simulink model "s2"  (Simulink 2.00)
settings: Solver=ode5  StartTime=0.0  StopTime=tstop  FixedStep=0.005  MaxStep=0.005  RelTol=1e-6  AbsTol=1e-6
values from neighbouring files (symbols this model uses):
  alpha = input('Enter attenuation factor, alpha > ')    [M2.M]    (also in M3.M = input('Enter attenuation factor alpha, try 1,  > '))
  m = input('Enter value of m  > ')    [M2.M]    (also in M3.M = input('Enter the value of m for abc currents  > '))
  n = input('Enter value of harmonic order n  > ')    [M2.M]
undefined symbols (not defined in the file or in its folder): sfunxy
settings Model: SaveTime=off  SaveOutput=off  ConsistencyChecking=off

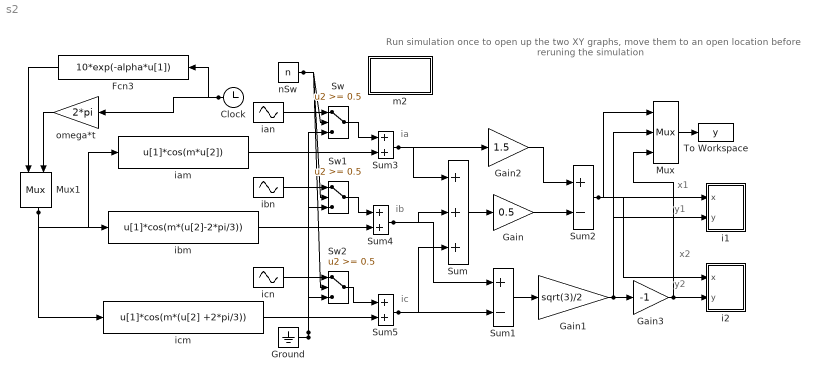
== system s2 ==
  note: ib
  note: ic
  note: x1
  note: x2
  note: y1
  note: y2
  note: ia
  note: Run simulation once to open up the two XY graphs, move
      | them to an open location before reruning  the simulation
  Clock : Clock
      settings: DeleteFcn=simclock BlockIsBeingDestroyed  PostSaveFcn=simclock Save
  Fcn3 : Fcn  Orientation=left  Expr=10*exp(-alpha*u[1])
  Gain : Gain  Gain=0.5
  Gain1 : Gain  Gain=sqrt(3)/2
  Gain2 : Gain  Gain=1.5
  Gain3 : Gain  Gain=-1
  Ground : Ground
  m2 : Subsystem
      settings: OpenFcn=m2
      mask Type: Masked block of m2.m
      mask Help: Uses m2.m to initialize and plot results
      mask Display: disp('Initialize\nand plot')
  Mux : Mux  Inputs=3
  Mux1 : Mux  Orientation=down  Inputs=2
  Sum : Sum  Inputs=+++
  Sum1 : Sum  Inputs=+-
  Sum2 : Sum  Inputs=+-
  Sum3 : Sum  Inputs=++
  Sum4 : Sum  Inputs=++
  Sum5 : Sum  Inputs=++
  Sw : Switch  Threshold=0.5
  Sw1 : Switch  Threshold=0.5
  Sw2 : Switch  Threshold=0.5
  To Workspace : ToWorkspace  VariableName=y  SampleTime=0
      settings: Buffer=1000
  i1 : Subsystem  mask(XY scope.){ax(1)=-20, ax(2)=20, ax(3)=-20, ax(4)=20, st=-1}
      mask prompts: ax(1) "x-min"; ax(2) "x-max"; ax(3) "y-min"; ax(4) "y-max"; st "Sample Time"
      mask help: XY scope using MATLAB graph window. First input is used as time base. Enter plotting ranges.
      mask Help: This block can be used to explore limit cycles. Look at the m-file sfunxy.m to see how it works.
      mask Display: plot([.05 .95 .95 .05 .05],[.45 .45 .95 .95 .45], 0.5+cos(0:0.1:2*pi)*0.3,0.7+sin(0:0.1:2*pi)*0.2)
  i2 : Subsystem  mask(XY scope.){ax(1)=-20, ax(2)=20, ax(3)=-20, ax(4)=20, st=-1}
      mask prompts: ax(1) "x-min"; ax(2) "x-max"; ax(3) "y-min"; ax(4) "y-max"; st "Sample Time"
      mask help: XY scope using MATLAB graph window. First input is used as time base. Enter plotting ranges.
      mask Help: This block can be used to explore limit cycles. Look at the m-file sfunxy.m to see how it works.
      mask Display: plot([.05 .95 .95 .05 .05],[.45 .45 .95 .95 .45], 0.5+cos(0:0.1:2*pi)*0.3,0.7+sin(0:0.1:2*pi)*0.2)
  iam : Fcn  Expr=u[1]*cos(m*u[2])
  ian : Sin  Amplitude=10/n  Frequency=(2*pi)*n  Phase=n*pi/2  SampleTime=-1
  ibm : Fcn  Expr=u[1]*cos(m*(u[2]-2*pi/3))
  ibn : Sin  Amplitude=10/n  Frequency=(2*pi)*n  Phase=-n*pi/6  SampleTime=-1
  icm : Fcn  Expr=u[1]*cos(m*(u[2] +2*pi/3))
  icn : Sin  Amplitude=10/n  Frequency=(2*pi)*n  Phase=n*7*pi/6  SampleTime=-1
  nSw : Constant  Value=n
  omega*t : Gain  Orientation=left  Gain=2*pi
  wires:
  Sum1/1 -> Gain1/1
  Sum/1 -> Gain/1
  Gain/1 -> Sum2/2
  Gain2/1 -> Sum2/1
  Sum2/1 -> i1/1(x), i2/1(x), Mux/1
  Gain1/1 -> i1/2(y), Gain3/1, Mux/2
  Gain3/1 -> i2/2(y), Mux/3
  Mux/1 -> To Workspace/1
  Sum3/1 -> Gain2/1, Sum/1
  Sum5/1 -> Sum1/2, Sum/3
  Sum4/1 -> Sum/2, Sum1/1
  ian/1 -> Sw/1
  Sw/1 -> Sum3/1
  ibn/1 -> Sw1/1
  Sw1/1 -> Sum4/1
  icn/1 -> Sw2/1
  Sw2/1 -> Sum5/1
  nSw/1 -> Sw2/2, Sw1/2, Sw/2
  iam/1 -> Sum3/2
  ibm/1 -> Sum4/2
  icm/1 -> Sum5/2
  Fcn3/1 -> Mux1/1
  Clock/1 -> omega*t/1, Fcn3/1
  omega*t/1 -> Mux1/2
  Mux1/1 -> iam/1, ibm/1, icm/1
  Ground/1 -> Sw2/3, Sw/3, Sw1/3

== system s2/m2 ==
  note: Masked block m2.m
      | to initialize s2.m and plot results

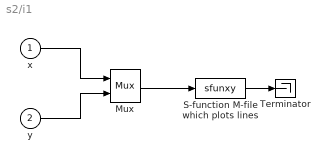
== system s2/i1 ==
  x : Inport  Port=1  PortWidth=-1  SampleTime=-1
  y : Inport  Port=2  PortWidth=-1  SampleTime=-1
  Mux : Mux  Inputs=2
  "S-function M-file which plots lines " : S-Function  LoadFcn=sfunxy([],[],[],'LoadBlock')  FunctionName=sfunxy  Parameters=ax, st
      settings: CopyFcn=sfunxy([],[],[],'CopyBlock')  DeleteFcn=sfunxy([],[],[],'DeleteBlock')
  Terminator : Terminator
  wires:
  "S-function M-file which plots lines "/1 -> Terminator/1
  y/1 -> Mux/2
  x/1 -> Mux/1
  Mux/1 -> "S-function M-file which plots lines "/1

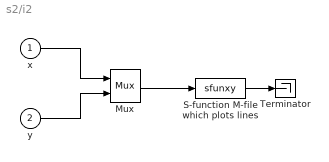
== system s2/i2 ==
  x : Inport  Port=1  PortWidth=-1  SampleTime=-1
  y : Inport  Port=2  PortWidth=-1  SampleTime=-1
  Mux : Mux  Inputs=2
  "S-function M-file which plots lines " : S-Function  LoadFcn=sfunxy([],[],[],'LoadBlock')  FunctionName=sfunxy  Parameters=ax, st
      settings: CopyFcn=sfunxy([],[],[],'CopyBlock')  DeleteFcn=sfunxy([],[],[],'DeleteBlock')
  Terminator : Terminator
  wires:
  "S-function M-file which plots lines "/1 -> Terminator/1
  y/1 -> Mux/2
  x/1 -> Mux/1
  Mux/1 -> "S-function M-file which plots lines "/1
